simulink model "testpso2"  (R2021a)
settings: Solver=VariableStepAuto  StartTime=0.0  StopTime=60  RelTol=1e-3
undefined symbols (not defined in the file or in its folder): kk, sigbuilder_block
settings Model: Creator=uddin  LastModifiedBy=uddin

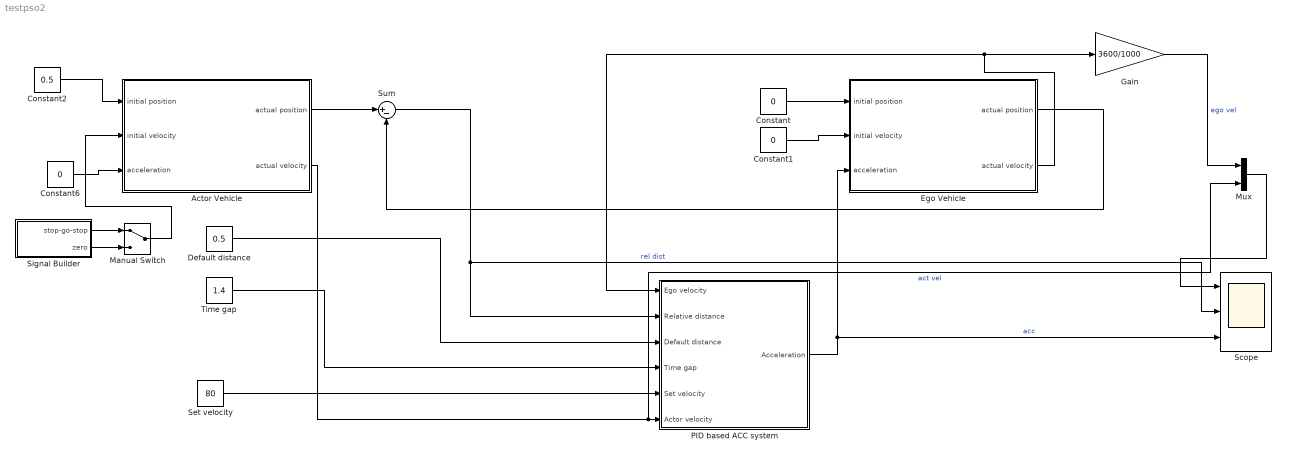
== system testpso2 ==
  Actor Vehicle : Subsystem
  Constant : Constant  Value=0  SampleTime=.1
  Constant1 : Constant  Value=0  SampleTime=.1
  Constant2 : Constant  Value=0.5  SampleTime=.1
  Constant6 : Constant  Value=0  SampleTime=.1
  Default distance : Constant  Value=0.5  SampleTime=.1
  Ego Vehicle : Subsystem
  Gain : Gain  Gain=3600/1000
  Manual Switch : ManualSwitch
  Mux : Mux  Inputs=2
  PID based ACC system : Subsystem
  Scope : Scope  NumInputPorts=3
  Set velocity : Constant  Value=80  SampleTime=.1
  Signal Builder : Subsystem  Tag=STV Subsys  LoadFcn=sigbuilder_block('load');  StartFcn=sigbuilder_block('start');  StopFcn=sigbuilder_block('stop');  ClipboardFcn=sigbuilder_block('clipboard');  mask(Sigbuilder block){tuvar=[0:10]}
      mask help: Simulink:masks:SigbuilderBlock_MD
      mask init:
      | if ~strcmp(get_param(bdroot(gcbh),'SimulationStatus'),'stopped') tuvar = sigbuilder_block('maskInit'); end
      settings: CopyFcn=sigbuilder_block('copy');  DeleteFcn=sigbuilder_block('delete');  ModelCloseFcn=sigbuilder_block('modelClose');  PreSaveFcn=sigbuilder_block('preSave');  PauseFcn=sigbuilder_block('pause');  ContinueFcn=sigbuilder_block('continue');  NameChangeFcn=sigbuilder_block('namechange');  OpenFcn=sigbuilder_block('open',[393 134.4 550.8 400.2 ]);  CloseFcn=sigbuilder_block('close');
      mask Display: plot(0, 0, 100, 100,[2, 2, 32, 32, 2], [68, 8, 8, 68, 68],[32, 2], [38, 38], [32, 19, 2],[53, 60, 44], [32, 17, 17, 2],[16, 16, 31, 31]);txt = getActiveGroup(gcbh);text(2, 100, txt,'verticalAlignment', 'top');
  Sum : Sum  Inputs=|+-
  Time gap : Constant  Value=1.4  SampleTime=.1
  wires:
  Ego Vehicle/2(actual velocity) -> PID based ACC system/1(Ego velocity), Gain/1
  Set velocity/1 -> PID based ACC system/5(Set velocity)
  Constant6/1 -> Actor Vehicle/3(acceleration)
  Sum/1 -> PID based ACC system/2(Relative distance), Scope/2  "rel dist"
  Time gap/1 -> PID based ACC system/4(Time gap)
  PID based ACC system/1(Acceleration) -> Ego Vehicle/3(acceleration), Scope/3  "acc"
  Actor Vehicle/2(actual velocity) -> Mux/2, PID based ACC system/6(Actor velocity)  "act vel"
  Gain/1 -> Mux/1  "ego vel"
  Ego Vehicle/1(actual position) -> Sum/2
  Constant2/1 -> Actor Vehicle/1(initial position)
  Constant1/1 -> Ego Vehicle/2(initial velocity)
  Actor Vehicle/1(actual position) -> Sum/1
  Constant/1 -> Ego Vehicle/1(initial position)
  Default distance/1 -> PID based ACC system/3(Default distance)
  Mux/1 -> Scope/1
  Signal Builder/1(stop-go-stop) -> Manual Switch/1
  Signal Builder/2(zero) -> Manual Switch/2
  Manual Switch/1 -> Actor Vehicle/2(initial velocity)

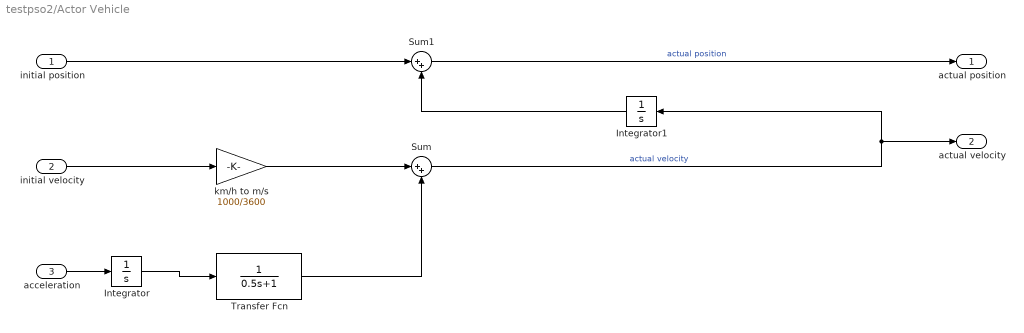
== system testpso2/Actor Vehicle ==
  initial position : Inport
  initial velocity : Inport  Port=2
  acceleration : Inport  Port=3
  Integrator : Integrator
  Integrator1 : Integrator
  Sum : Sum  Inputs=|++
  Sum1 : Sum  Inputs=|++
  Transfer Fcn : TransferFcn  Denominator=[0.5 1]
  km/h to m/s : Gain  Gain=1000/3600
  actual position : Outport
  actual velocity : Outport  Port=2
  wires:
  km/h to m/s/1 -> Sum/1
  initial velocity/1 -> km/h to m/s/1
  Transfer Fcn/1 -> Sum/2
  Integrator/1 -> Transfer Fcn/1
  Integrator1/1 -> Sum1/2
  initial position/1 -> Sum1/1
  acceleration/1 -> Integrator/1
  Sum/1 -> Integrator1/1, actual velocity/1  "actual velocity"
  Sum1/1 -> actual position/1  "actual position"

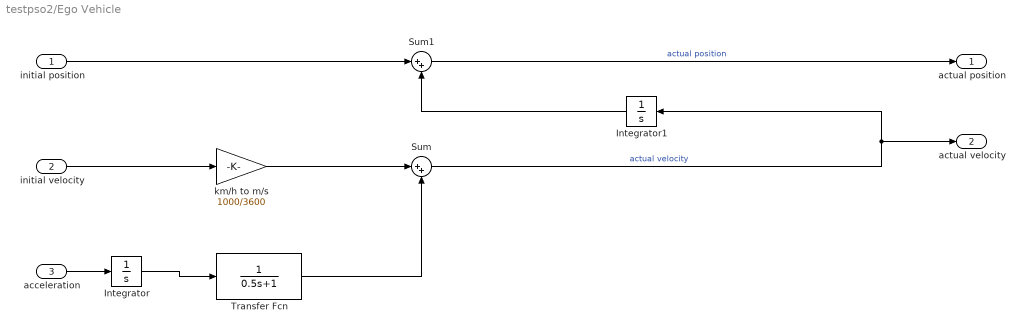
== system testpso2/Ego Vehicle ==
  initial position : Inport
  initial velocity : Inport  Port=2
  acceleration : Inport  Port=3
  Integrator : Integrator
  Integrator1 : Integrator
  Sum : Sum  Inputs=|++
  Sum1 : Sum  Inputs=|++
  Transfer Fcn : TransferFcn  Denominator=[0.5 1]
  km/h to m/s : Gain  Gain=1000/3600
  actual position : Outport
  actual velocity : Outport  Port=2
  wires:
  Sum1/1 -> actual position/1  "actual position"
  Sum/1 -> actual velocity/1, Integrator1/1  "actual velocity"
  acceleration/1 -> Integrator/1
  initial position/1 -> Sum1/1
  Integrator1/1 -> Sum1/2
  Integrator/1 -> Transfer Fcn/1
  Transfer Fcn/1 -> Sum/2
  initial velocity/1 -> km/h to m/s/1
  km/h to m/s/1 -> Sum/1

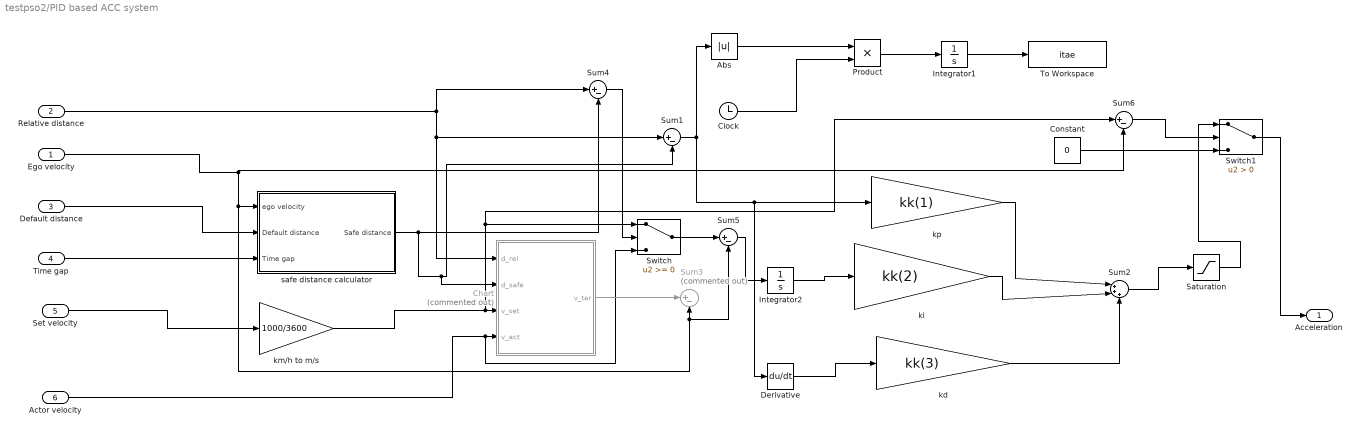
== system testpso2/PID based ACC system ==
  Ego velocity : Inport
  Relative distance : Inport  Port=2
  Default distance : Inport  Port=3
  Time gap : Inport  Port=4
  Set velocity : Inport  Port=5
  Actor velocity : Inport  Port=6
  Abs : Abs  ZeroCross=off
  Chart : Stateflow chart  Commented=on  TreatAsAtomicUnit=on
  Clock : Clock
  Constant : Constant  Value=0  SampleTime=0.1
  Derivative : Derivative
  Integrator1 : Integrator
  Integrator2 : Integrator
  Product : Product
  Saturation : Saturate  UpperLimit=2  LowerLimit=-3  LinearizeAsGain=off  ZeroCross=off
  Sum{1,4..6} (4 alike) : Sum  Inputs=|+-
  Sum2 : Sum  Inputs=|+++
  Sum3 : Sum  Commented=on  Inputs=|+-
  Switch : Switch  ZeroCross=off
  Switch1 : Switch  Criteria=u2 > Threshold  ZeroCross=off
  To Workspace : ToWorkspace  VariableName=itae  SampleTime=1
      settings: Save2DSignal=2-D array (concatenate along first dimension)
  kd : Gain  Gain=kk(3)
  ki : Gain  Gain=kk(2)
  km/h to m/s : Gain  Gain=1000/3600
  kp : Gain  Gain=kk(1)
  safe distance calculator : Subsystem
  Acceleration : Outport
  wires:
  Default distance/1 -> safe distance calculator/2(Default distance)
  Set velocity/1 -> km/h to m/s/1
  Time gap/1 -> safe distance calculator/3(Time gap)
  Ego velocity/1 -> Sum6/2, safe distance calculator/1(ego velocity), Sum5/2, Sum3/2
  ki/1 -> Sum2/2
  kp/1 -> Sum2/1
  Relative distance/1 -> Sum4/1, Chart/1(d_rel), Sum1/1
  safe distance calculator/1(Safe distance) -> Sum4/2, Sum1/2, Chart/2(d_safe)
  km/h to m/s/1 -> Switch/1, Sum6/1, Chart/3(v_set)
  Actor velocity/1 -> Switch/3, Chart/4(v_act)
  Sum1/1 -> Derivative/1, kp/1, Abs/1
  Abs/1 -> Product/1
  Derivative/1 -> kd/1
  kd/1 -> Sum2/3
  Chart/1(v_tar) -> Sum3/1
  Integrator2/1 -> ki/1
  Sum2/1 -> Saturation/1
  Product/1 -> Integrator1/1
  Integrator1/1 -> To Workspace/1
  Clock/1 -> Product/2
  Sum4/1 -> Switch/2
  Switch/1 -> Sum5/1
  Sum5/1 -> Integrator2/1
  Constant/1 -> Switch1/3
  Switch1/1 -> Acceleration/1
  Saturation/1 -> Switch1/1
  Sum6/1 -> Switch1/2

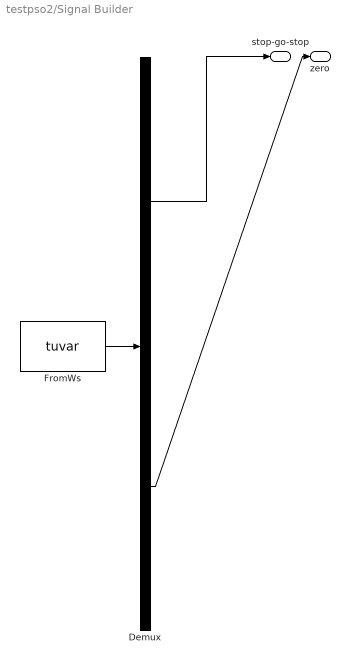
== system testpso2/Signal Builder ==
  Demux : Demux  Tag=STV Demux  Outputs=2
      settings: DisplayOption=none
  FromWs : FromWorkspace  Tag=STV FromWs  VariableName=tuvar
      SigBuilderData=|
      | common.afterFinalStr = 'Extrapolate'
      | common.sampleTime = 0
      | dataSet.timeRange = [0 30]
      | dataSet.name = 'Group 1'
      | sbobj.Groups.Name = 'Group 1'
      | sbobj.Groups.Signals(1).Name = 'stop-go-stop'
      | sbobj.Groups.Signals(1).XData = [0 5 10 20 25 30]
      | sbobj.Groups.Signals(1).YData = [0 0 2 2 0 0]
      | sbobj.Groups.Signals(2).Name = 'zero'
      | sbobj.Groups.Signals(2).XData = [0 30]
      | sbobj.Groups.Signals(2).YData = [0 0]
      | sbobj.Groups.TimeRange = [0 30]
  stop-go-stop : Outport  Tag=STV Outport
  zero : Outport  Tag=STV Outport  Port=2
  wires:
  FromWs/1 -> Demux/1
  Demux/1 -> stop-go-stop/1
  Demux/2 -> zero/1

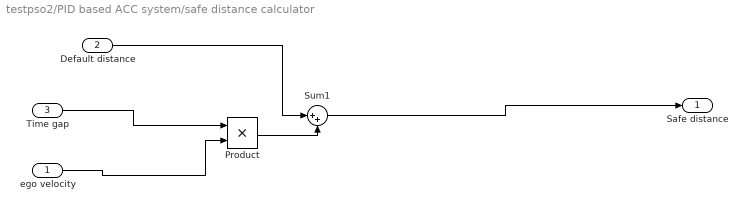
== system testpso2/PID based ACC system/safe distance calculator ==
  ego velocity : Inport
  Default distance : Inport  Port=2
  Time gap : Inport  Port=3
  Product : Product
  Sum1 : Sum  Inputs=|++
  Safe distance : Outport
  wires:
  Product/1 -> Sum1/2
  Sum1/1 -> Safe distance/1
  Time gap/1 -> Product/1
  Default distance/1 -> Sum1/1
  ego velocity/1 -> Product/2

== stateflow chart testpso2/PID based ACC system/Chart ==
  (default) -> (junction 7)
  (junction 7) -> (junction 8) [order 1] : [d_rel>d_safe]
  (junction 7) -> (junction 9) [order 2] : {v_tar=v_act;}
  (junction 8) -> (junction 10) : {v_tar=v_set;}
  (junction 10) -> (junction 9)
  (junction 9) -> (junction 11)
  data: d_rel input; d_safe input; v_set input; v_act input; v_tar output
